simulink model "trafficstateflow"  (R2016a)
settings: Solver=FixedStepDiscrete  StartTime=0.0  StopTime=inf  RelTol=1e-3
settings Model: Creator=yasme  LastModifiedBy=yasme
settings OptimizationCC: DefaultParameterBehavior=Inlined  OptimizeModelRefInitCode=on  LifeSpan=1
settings DebuggingCC: UnderspecifiedInitializationDetection=Classic  MergeDetectMultiDrivingBlocksExec=none
settings ModelReferenceCC: PropagateSignalLabelsOutOfModel=off
settings RTWCC: SystemTargetFile=ert.tlc  GenCodeOnly=on  TemplateMakefile=ert_default_tmf  GenerateReport=on  IncludeHyperlinkInReport=on  LaunchReport=on  GenerateTraceInfo=on  GenerateTraceReport=on  GenerateTraceReportSl=on  GenerateTraceReportSf=on  GenerateTraceReportEml=on
settings CodeAppCC: ForceParamTrailComments=on  IgnoreCustomStorageClasses=off  OperatorAnnotations=on  SimulinkDataObjDesc=on  SFDataObjDesc=on  MATLABFcnDesc=on  InsertBlockDesc=on  MATLABSourceComments=on
settings ERTTargetCC: GenerateSampleERTMain=on  InlinedParameterPlacement=NonHierarchical  ERTCustomFileTemplate=example_file_process.tlc

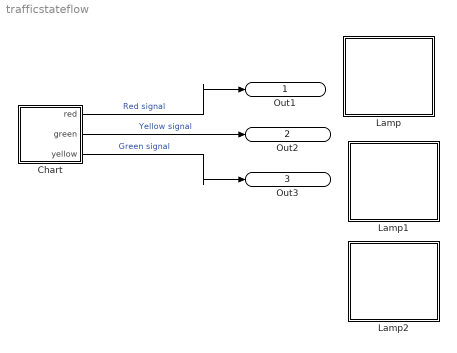
== system trafficstateflow ==
  Chart : Stateflow chart  TreatAsAtomicUnit=on
  Lamp : Subsystem  DialogController=hmiCreateDDGDialog  IsWebBlock=on  mask(MWDashboardBlock){webBlockId=b4a4c831-9db9-49b5-802a-d5744f73d539, webBlockType=lamp, ShowInLibBrowser=on, ShowInitialText=on, HMISrcModelName=trafficstateflow}
      mask prompts: webBlockType "WebBlock Type"; HMISrcModelName "Source Model"
      mask Help: helpview([docroot '/mapfiles/simulink.map'], 'hmi_lamp')
      mask Display:
      | if strcmp(get_param(bdroot(gcb),'BlockDiagramType'), 'library')
      |     image([(matlabroot) '/toolbox/simulink/hmi/icons/Lamp.png']);
      | end
  Lamp1 : Subsystem  DialogController=hmiCreateDDGDialog  IsWebBlock=on  mask(MWDashboardBlock){webBlockId=575b6775-f35a-4be6-8dde-81a9fe826c5b, webBlockType=lamp, ShowInLibBrowser=on, ShowInitialText=on, HMISrcModelName=trafficstateflow}
      mask prompts: webBlockType "WebBlock Type"; HMISrcModelName "Source Model"
      mask Help: helpview([docroot '/mapfiles/simulink.map'], 'hmi_lamp')
      mask Display:
      | if strcmp(get_param(bdroot(gcb),'BlockDiagramType'), 'library')
      |     image([(matlabroot) '/toolbox/simulink/hmi/icons/Lamp.png']);
      | end
  Lamp2 : Subsystem  DialogController=hmiCreateDDGDialog  IsWebBlock=on  mask(MWDashboardBlock){webBlockId=9ff9998b-57a1-4d2e-8163-c8b9ff2d12cc, webBlockType=lamp, ShowInLibBrowser=on, ShowInitialText=on, HMISrcModelName=trafficstateflow}
      mask prompts: webBlockType "WebBlock Type"; HMISrcModelName "Source Model"
      mask Help: helpview([docroot '/mapfiles/simulink.map'], 'hmi_lamp')
      mask Display:
      | if strcmp(get_param(bdroot(gcb),'BlockDiagramType'), 'library')
      |     image([(matlabroot) '/toolbox/simulink/hmi/icons/Lamp.png']);
      | end
  Out1 : Outport  OutDataTypeStr=uint8
  Out2 : Outport  Port=2  OutDataTypeStr=uint8
  Out3 : Outport  Port=3  OutDataTypeStr=uint8
  wires:
  Chart/1(red) -> Out1/1  "Red signal"
  Chart/2(green) -> Out2/1  "Yellow signal"
  Chart/3(yellow) -> Out3/1  "Green signal"

== system trafficstateflow/Lamp ==

== system trafficstateflow/Lamp1 ==

== system trafficstateflow/Lamp2 ==

== stateflow chart trafficstateflow/Chart ==
  state Stop_
    en:
    red=uint8(0);
    green=uint8(0);
    du:
    red=uint8(1);
    yellow=uint8(0);
    green=uint8(0);
    ex:
  state Ready_
    en:
    red=uint8(0);
    green=uint8(0);
    du:
    red=uint8(0);
    yellow=uint8(1);
    green=uint8(0);
    ex:
  state Green_
    en:
    red=uint8(0);
    green=uint8(0);
    du:
    red=uint8(0);
    yellow=uint8(0);
    green=uint8(1);
    ex:
  Stop_ -> Ready_ : after(3000,msec)
  (default) -> Stop_
  Green_ -> Stop_ : after(3000,msec)
  Ready_ -> Green_ : after(3000,msec)
  data: red output uint8; green output uint8; yellow output uint8
